simulink model "MCU_CmdTrans"  (R2022b)
settings: Solver=FixedStepDiscrete  StartTime=0.0  StopTime=10.0  FixedStep=0.001  RelTol=1e-3
undefined symbols (not defined in the file or in its folder): ANALOG, cAgeingMode, cCurrentLoopMode, cNoneMode, cParaRecogMode, cSingleBoardMode, cSpeedLoopMode, cTorqueLoopMode, cVvvfOpenMode, FAULT, ParamCfg_CommandSource_u16, ParamCfg_MaxSpeed_u16, ParamCfg_MaxTorque_u16, ParamCfg_Spdouttype_u16, ParamCfg_Vc1Enable_u16, POWER_ON, STANDBY, TESTBED, VEHICLE, WORKING
libraries: simulink x9
(part 2 of 2)

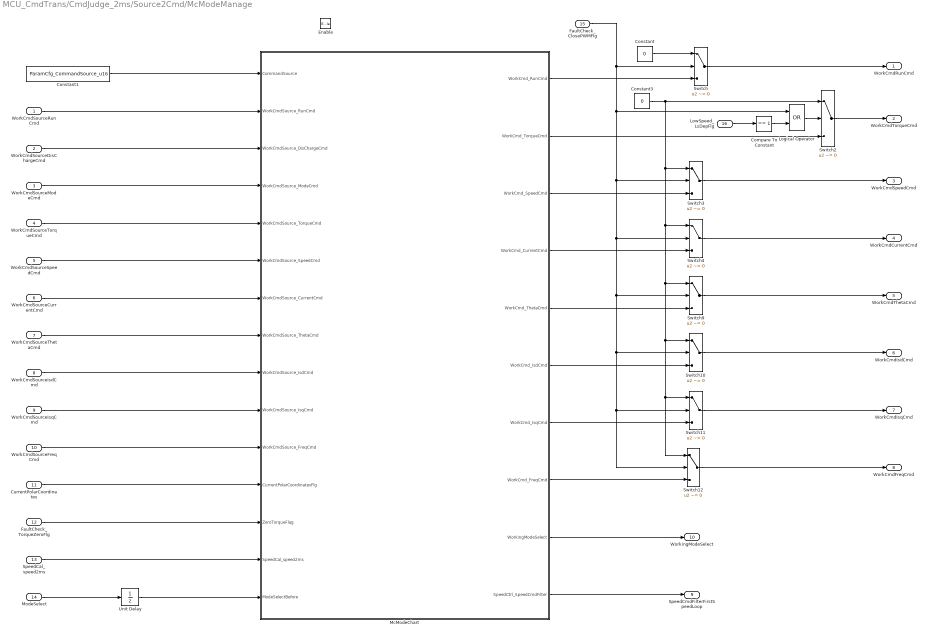
== system MCU_CmdTrans/CmdJudge_2ms/Source2Cmd/McModeManage ==
  WorkCmdSourceRunCmd : Inport
  WorkCmdSourceDisChargeCmd : Inport  Port=2
  WorkCmdSourceModeCmd : Inport  Port=3
  WorkCmdSourceTorqueCmd : Inport  Port=4
  WorkCmdSourceSpeedCmd : Inport  Port=5
  WorkCmdSourceCurrentCmd : Inport  Port=6
  WorkCmdSourceThetaCmd : Inport  Port=7
  WorkCmdSourceIsdCmd : Inport  Port=8
  WorkCmdSourceIsqCmd : Inport  Port=9
  WorkCmdSourceFreqCmd : Inport  Port=10
  CurrentPolarCoordinates : Inport  Port=11
  FaultCheck_TorqueZeroFlg : Inport  Port=12
  SpeedCal_speed2ms : Inport  Port=13
  ModeSelect : Inport  Port=14
  FaultCheck_ClosePWMFlg : Inport  Port=15
  LowSpeed_LsDepFlg : Inport  Port=16
  Enable : EnablePort
  Compare To Constant : simulink/Logic and Bit Operations/Compare To Constant  relop===  const=1  OutDataTypeStr=boolean
  Constant : Constant  Value=0  OutDataTypeStr=uint16
  Constant1 : Constant  Value=ParamCfg_CommandSource_u16
  Constant3 : Constant  Value=0  OutDataTypeStr=single
  Logical Operator : Logic  Operator=OR  AllPortsSameDT=off  OutDataTypeStr=boolean
  McModeChart : Stateflow chart  TreatAsAtomicUnit=on
      settings: FunctionInterfaceSpec=Allow arguments (Optimized)  PortSchema="{\"entries\":[{\"content\":{\"sides\":[{\"content\":{\"connectorIds\":[\"In2\",\"In5\",\"In3\",\"In4\",\"In6\",\"In11\",\"In7\",\"In1\",\"In9\",\"In10\",\"In8\",\"In12\",\"In13\",\"In14\",\"In15\"]},\"type\":\"ConnectorPlacement.EquallySpacedRectSide\",\"uuid\":\"2e7d3842-0a61-4590-9292-7a5bc1b6d63e\"},{\"content\":{\"connectorIds\":[\"Out2\",\"Out3\",\"Out4\",\"Out6\",\"Out5\",\"Out7\",\"Out8\",\"Out9\",\"Out1\",\"Out10\"],\"side\":\"RIGHT\"},\"type\":\"ConnectorPlacement.EquallySpacedRectSide\",\"uuid\":\"fb66f02a-321f-47a6-a489-4b94442e22c8\"},{\"content\":{\"connectorIds\":[],\"side\":\"TOP\"},\"type\":\"ConnectorPlacement.EquallySpacedRectSide\",\"uuid\":\"26cfdcf8-827e-48d9-aa42-40739db869be\"},{\"content\":{\"connectorIds\":[],\"side\":\"BOTTOM\"},\"type\":\"ConnectorPlacement.EquallySpacedRectSide\",\"uuid\":\"3bc2be8d-756f-48d1-976e-919451ea6fa2\"}]},\"type\":\"ConnectorPlacement.EquallySpacedConnector\",\"uuid\":\"eb156a25-beb1-4594-a414-e9203ec852c3\"}],\"packageUris\":[\"http://schema.mathworks.com/mf0/Connector/R2020b\"],\"version\":\"1.0\"}"
  Switch{,2..4,9..12} (8 alike) : Switch  Criteria=u2 ~= 0  SaturateOnIntegerOverflow=off  InputSameDT=off
  Unit Delay : UnitDelay  SampleTime=-1  HasFrameUpgradeWarning=on
  WorkCmdRunCmd : Outport
  WorkCmdTorqueCmd : Outport  Port=2
  WorkCmdSpeedCmd : Outport  Port=3
  WorkCmdCurrentCmd : Outport  Port=4
  WorkCmdThetaCmd : Outport  Port=5
  WorkCmdIsdCmd : Outport  Port=6
  WorkCmdIsqCmd : Outport  Port=7
  WorkCmdFreqCmd : Outport  Port=8
  SpeedCmdFilterFirstSpeedLoop : Outport  Port=9
  WorkingModeSelect : Outport  Port=10
  wires:
  Constant1/1 -> McModeChart/2(CommandSource)
  WorkCmdSourceRunCmd/1 -> McModeChart/5(WorkCmdSource_RunCmd)
  WorkCmdSourceModeCmd/1 -> McModeChart/4(WorkCmdSource_ModeCmd)
  WorkCmdSourceTorqueCmd/1 -> McModeChart/6(WorkCmdSource_TorqueCmd)
  WorkCmdSourceDisChargeCmd/1 -> McModeChart/3(WorkCmdSource_DisChargeCmd)
  WorkCmdSourceSpeedCmd/1 -> McModeChart/11(WorkCmdSource_SpeedCmd)
  WorkCmdSourceCurrentCmd/1 -> McModeChart/7(WorkCmdSource_CurrentCmd)
  WorkCmdSourceThetaCmd/1 -> McModeChart/1(WorkCmdSource_ThetaCmd)
  WorkCmdSourceIsdCmd/1 -> McModeChart/9(WorkCmdSource_IsdCmd)
  WorkCmdSourceIsqCmd/1 -> McModeChart/10(WorkCmdSource_IsqCmd)
  WorkCmdSourceFreqCmd/1 -> McModeChart/8(WorkCmdSource_FreqCmd)
  CurrentPolarCoordinates/1 -> McModeChart/12(CurrentPolarCoordinatesFlg)
  FaultCheck_TorqueZeroFlg/1 -> McModeChart/13(ZeroTorqueFlag)
  SpeedCal_speed2ms/1 -> McModeChart/14(SpeedCal_speed2ms)
  ModeSelect/1 -> Unit Delay/1
  Unit Delay/1 -> McModeChart/15(ModeSelectBefore)
  FaultCheck_ClosePWMFlg/1 -> Switch12/2, Switch11/2, Switch10/2, Switch9/2, Switch4/2, Switch3/2, Logical Operator/1, Switch/2
  McModeChart/2(WorkCmd_RunCmd) -> Switch/3
  Constant/1 -> Switch/1
  McModeChart/3(WorkCmd_TorqueCmd) -> Switch2/3
  Constant3/1 -> Switch12/1, Switch11/1, Switch10/1, Switch9/1, Switch4/1, Switch3/1, Switch2/1
  McModeChart/4(WorkCmd_SpeedCmd) -> Switch3/3
  McModeChart/6(WorkCmd_CurrentCmd) -> Switch4/3
  McModeChart/5(WorkCmd_ThetaCmd) -> Switch9/3
  McModeChart/7(WorkCmd_IsdCmd) -> Switch10/3
  McModeChart/8(WorkCmd_IsqCmd) -> Switch11/3
  McModeChart/9(WorkCmd_FreqCmd) -> Switch12/3
  McModeChart/10(SpeedCtrl_SpeedCmdFilter) -> SpeedCmdFilterFirstSpeedLoop/1
  Switch/1 -> WorkCmdRunCmd/1
  Switch2/1 -> WorkCmdTorqueCmd/1
  Switch3/1 -> WorkCmdSpeedCmd/1
  Switch4/1 -> WorkCmdCurrentCmd/1
  Switch9/1 -> WorkCmdThetaCmd/1
  Switch10/1 -> WorkCmdIsdCmd/1
  Switch11/1 -> WorkCmdIsqCmd/1
  Switch12/1 -> WorkCmdFreqCmd/1
  McModeChart/1(WorkingModeSelect) -> WorkingModeSelect/1
  LowSpeed_LsDepFlg/1 -> Compare To Constant/1
  Logical Operator/1 -> Switch2/2
  Compare To Constant/1 -> Logical Operator/2

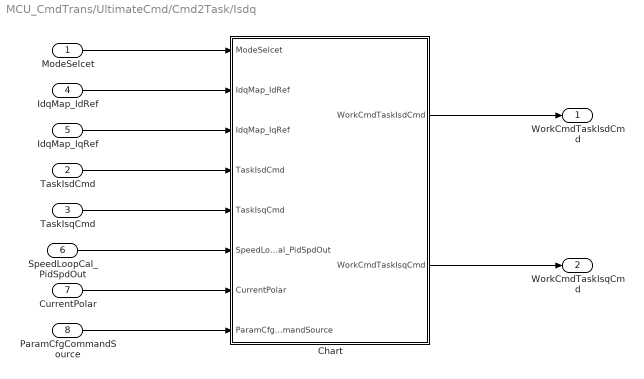
== system MCU_CmdTrans/UltimateCmd/Cmd2Task/Isdq ==
  ModeSelcet : Inport
  TaskIsdCmd : Inport  Port=2
  TaskIsqCmd : Inport  Port=3
  IdqMap_IdRef : Inport  Port=4
  IdqMap_IqRef : Inport  Port=5
  SpeedLoopCal_PidSpdOut : Inport  Port=6
  CurrentPolar : Inport  Port=7
  ParamCfgCommandSource : Inport  Port=8
  Chart : Stateflow chart  TreatAsAtomicUnit=on
  WorkCmdTaskIsdCmd : Outport
  WorkCmdTaskIsqCmd : Outport  Port=2
  wires:
  ModeSelcet/1 -> Chart/1(ModeSelcet)
  IdqMap_IdRef/1 -> Chart/2(IdqMap_IdRef)
  TaskIsdCmd/1 -> Chart/4(TaskIsdCmd)
  IdqMap_IqRef/1 -> Chart/3(IdqMap_IqRef)
  TaskIsqCmd/1 -> Chart/5(TaskIsqCmd)
  Chart/1(WorkCmdTaskIsdCmd) -> WorkCmdTaskIsdCmd/1
  Chart/2(WorkCmdTaskIsqCmd) -> WorkCmdTaskIsqCmd/1
  SpeedLoopCal_PidSpdOut/1 -> Chart/6(SpeedLoopCal_PidSpdOut)
  CurrentPolar/1 -> Chart/7(CurrentPolar)
  ParamCfgCommandSource/1 -> Chart/8(ParamCfgCommandSource)

== stateflow chart MCU_CmdTrans/UltimateCmd/Cmd2Task/Cmd2TaskChart ==
  (default) -> (junction 18)
  (junction 18) -> (junction 20) [order 1] : [WorkState_ModeSelect ==cTorqueLoopMode]
  (junction 18) -> (junction 50) [order 2]
  (junction 20) -> (junction 22) : {
      | WorkCmdTaskRunCmd = WorkCmdRunCmd;
      | WorkCmdTaskTorqueCmd = WorkCmdTorqueCmd;
      | }
  (junction 28) -> (junction 32) [order 1] : [(SpeedCal_HighSpdZeroTrqFlg == 0)&&(TorqeCtrl_TorqueCmdFilterAbs<0.001 && WorkCmdTaskTorqueCmd < 0.001)]{WorkCmdTaskRunCmd = STOP}
  (junction 22) -> (junction 25) [order 1] : [WorkCmdTaskTorqueCmd > 0]{SpeedCmdDir =1}
  (junction 22) -> (junction 25) [order 2] : {SpeedCmdDir = -1}
  (junction 25) -> (junction 28) : {WorkCmdTaskSpeedCmd = ParamCfg_MaxSpeed_u16 * SpeedCmdDir}
  (junction 28) -> (junction 32) [order 2]
  (junction 32) -> (junction 58)
  (junction 50) -> (junction 52) [order 1] : [WorkState_ModeSelect == cSpeedLoopMode]
  (junction 50) -> (junction 61) [order 2]
  (junction 52) -> (junction 54) : {WorkCmdTaskRunCmd = WorkCmdRunCmd;
      | WorkCmdTaskSpeedCmd = WorkCmdSpeedCmd;
      | WorkCmdTaskTorqueCmd = (ParamCfg_MaxTorque_u16 * 0.1)}
  (junction 54) -> (junction 58)
  (junction 58) -> (junction 67)
  (junction 61) -> (junction 63) [order 1] : [WorkState_ModeSelect == cCurrentLoopMode ]
  (junction 61) -> (junction 78) [order 2]
  (junction 63) -> (junction 65) : {WorkCmdTaskRunCmd = WorkCmdRunCmd}
  (junction 71) -> (junction 67) [order 1] : [(CurrentPolar == 1)&&ParamCfg_CommandSource_u16 == TESTBED]...
      | {WorkCmdTaskCurrentCmd = WorkCmdCurrentCmd;
      | WorkCmdTaskThetaCmd = WorkCmdThetaCmd;
      | WorkCmdTaskIsdCmd = WorkCmdTaskCurrentCmd * cos(WorkCmdTaskThetaCmd)*(-1)
      | WorkCmdTaskIsqCmd = WorkCmdTaskCurrentCmd * sin(WorkCmdTaskThetaCmd)
      | }
  (junction 71) -> (junction 67) [order 2] : {WorkCmdTaskIsdCmd = WorkCmdIsdCmd;
      | WorkCmdTaskIsqCmd = WorkCmdIsqCmd}
  (junction 65) -> (junction 71)
  (junction 67) -> (junction 85)
  (junction 78) -> (junction 80) [order 1] : [WorkState_ModeSelect == cVvvfOpenMode ]
  (junction 78) -> (junction 88) [order 2]
  (junction 80) -> (junction 83) : {WorkCmdTaskRunCmd = WorkCmdRunCmd;
      | WorkCmdTaskIsdCmd = WorkCmdIsdCmd;
      | WorkCmdTaskIsqCmd = WorkCmdIsqCmd;
      | WorkCmdTaskFreqCmd = WorkCmdFreqCmd;
      | }
  (junction 83) -> (junction 85)
  (junction 85) -> (junction 95)
  (junction 88) -> (junction 90) [order 1] : [WorkState_ModeSelect == cParaRecogMode ]
  (junction 88) -> (junction 98) [order 2]
  (junction 90) -> (junction 93) : {WorkCmdTaskRunCmd = WorkCmdRunCmd;
      | WorkCmdTaskRunCmd = WorkCmdRunCmd;
      | WorkCmdTaskIsdCmd = WorkCmdIsdCmd;
      | WorkCmdTaskIsqCmd = WorkCmdIsqCmd}
  (junction 93) -> (junction 95)
  (junction 95) -> (junction 105)
  (junction 98) -> (junction 100) [order 1] : [WorkState_ModeSelect == cSingleBoardMode ]
  (junction 98) -> (junction 108) [order 2]
  (junction 100) -> (junction 103) : {WorkCmdTaskRunCmd = WorkCmdRunCmd}
  (junction 103) -> (junction 105)
  (junction 105) -> (junction 125)
  (junction 108) -> (junction 110) [order 1] : [WorkState_ModeSelect == cAgeingMode ]
  (junction 108) -> (junction 112) [order 2]
  (junction 110) -> (junction 118) : {WorkCmdTaskRunCmd     = WorkCmdRunCmd;
      |  WorkCmdTaskCurrentCmd = (WorkCmdCurrentCmd);
      | WorkCmdTaskThetaCmd   = WorkCmdThetaCmd;
      |  WorkCmdTaskIsdCmd     = (WorkCmdTaskCurrentCmd * cos(WorkCmdTaskThetaCmd*2*PI));
      |  WorkCmdTaskIsqCmd     = (WorkCmdTaskCurrentCmd * sin(WorkCmdTaskThetaCmd*2*PI));
      |   WorkCmdTaskFreqCmd    = WorkCmdFreqCmd;}
  (junction 118) -> (junction 125)
  (junction 125) -> (junction 122)
  (junction 112) -> (junction 114) [order 1] : [WorkState_ModeSelect == cNoneMode ]
  (junction 112) -> (junction 129) [order 2]
  (junction 114) -> (junction 120) : {WorkCmdTaskRunCmd = STOP}
  (junction 120) -> (junction 122)
  (junction 122) -> (junction 131)
  (junction 131) -> (junction 129)
  (junction 129) -> (junction 134)
  data: WorkCmdIsdCmd input; WorkState_ModeSelect input; WorkCmdRunCmd input; WorkCmdTorqueCmd input; WorkCmdSpeedCmd input; WorkCmdCurrentCmd input; WorkCmdThetaCmd input; WorkCmdIsqCmd input; WorkCmdFreqCmd input; WorkCmdTaskRunCmd output uint16 =0; WorkCmdTaskTorqueCmd output single =0; WorkCmdTaskSpeedCmd output single =0; WorkCmdTaskCurrentCmd output single =0; WorkCmdTaskThetaCmd output single =0; WorkCmdTaskIsdCmd output single =0; WorkCmdTaskIsqCmd output single =0; WorkCmdTaskFreqCmd output single =0; cTorqueLoopMode parameter; SpeedCmdDir output double; SpeedCal_HighSpdZeroTrqFlg input; TorqeCtrl_TorqueCmdFilterAbs input; ParamCfg_MaxSpeed_u16 parameter; STOP constant uint16 =0; cSpeedLoopMode parameter; cCurrentLoopMode parameter; ParamCfg_MaxTorque_u16 parameter; CurrentPolar input; ParamCfg_CommandSource_u16 parameter; TESTBED parameter; cVvvfOpenMode parameter; cParaRecogMode parameter; cSingleBoardMode parameter; cAgeingMode parameter; cNoneMode parameter; PI constant single =3.141592

== stateflow chart MCU_CmdTrans/UltimateCmd/Cmd2Task/Isdq/Chart ==
  (default) -> (junction 8) : {
      | WorkCmdTaskIsdCmd = TaskIsdCmd;
      | WorkCmdTaskIsqCmd = TaskIsqCmd;
      | }
  (junction 8) -> (junction 10) [order 1] : [(ModeSelcet == cTorqueLoopMode) || (ModeSelcet==cSpeedLoopMode && ParamCfg_Spdouttype_u16 == 0)]
      | {WorkCmdTaskIsdCmd = IdqMap_IdRef;
      | WorkCmdTaskIsqCmd  = IdqMap_IqRef}
  (junction 8) -> (junction 10) [order 2]
  (junction 10) -> (junction 18) [order 1] : [ModeSelcet == cSpeedLoopMode &&ParamCfg_Spdouttype_u16 ==1 ]
      | {
      | WorkCmdTaskIsdCmd = 0;
      | WorkCmdTaskIsqCmd = SpeedLoopCal_PidSpdOut;
      | }
  (junction 10) -> (junction 18) [order 2]
  (junction 18) -> (junction 22) [order 1] : [ModeSelcet == cCurrentLoopMode && CurrentPolar == 1 && ParamCfgCommandSource == TESTBED]
      | {
      | WorkCmdTaskIsdCmd = 0;
      | WorkCmdTaskIsqCmd = SpeedLoopCal_PidSpdOut;
      | }
  (junction 18) -> (junction 22) [order 2]
  (junction 22) -> (junction 29)
  data: ModeSelcet input; IdqMap_IdRef input single; IdqMap_IqRef input single; TaskIsdCmd input; TaskIsqCmd input; WorkCmdTaskIsdCmd output; WorkCmdTaskIsqCmd output; cSpeedLoopMode parameter; cTorqueLoopMode parameter; ParamCfg_Spdouttype_u16 parameter; SpeedLoopCal_PidSpdOut input single; cCurrentLoopMode parameter; CurrentPolar input; ParamCfgCommandSource input; TESTBED parameter

== stateflow chart MCU_CmdTrans/CmdJudge_2ms/CAN2Source/Chart ==
  (default) -> (junction 26) : {
      | WorkCmdSourceRunCmd = RunCmd;
      | WorkCmdSourceDisChargeCmd = DisChargeCmd;
      | WorkCmdSourceModeCmd = ModeCmd;
      | WorkCmdSourceTorqueCmd = TorqueCmd;
      | WorkCmdSourceSpeedCmd = SpeedCmd;
      | WorkCmdSourceCurrentCmd = CurrentCmd;
      | WorkCmdSourceThetaCmd = ThetaCmd;
      | WorkCmdSourceIsdCmd = IsdCmd;
      | WorkCmdSourceIsqCmd = IsqCmd;
      | WorkCmdSourceFreqCmd = FreqCmd;
      | }
  (junction 26) -> (junction 28) [order 1] : [LsDepFlg == 1]{WorkCmdSourceTorqueCmd=0}
  (junction 26) -> (junction 28) [order 2]
  (junction 28) -> (junction 31) [order 1] : [FaultCheck_LostPhaseFaultFlg == 1]...
      | {WorkCmdSourceRunCmd = 1;
      | WorkCmdSourceModeCmd = cTorqueLoopMode}
  (junction 28) -> (junction 31) [order 2]
  (junction 31) -> (junction 35) [order 2] : [ActDisChargeStd == 1]...
      | {WorkCmdSourceRunCmd = 1;
      | WorkCmdSourceModeCmd = cCurrentLoopMode;
      | WorkCmdSourceIsdCmd = ActDisChargeCurr;
      | WorkCmdSourceIsqCmd = 0;
      | CurrentPolarCoordinates =0;}
  (junction 31) -> (junction 35) [order 1]
  (junction 35) -> (junction 40)
  data: RunCmd input; WorkCmdSourceRunCmd output uint16 =0; WorkCmdSourceDisChargeCmd output uint16 =0; WorkCmdSourceModeCmd output uint16 =0; WorkCmdSourceTorqueCmd output single =0; WorkCmdSourceSpeedCmd output single =0; WorkCmdSourceCurrentCmd output single =0; WorkCmdSourceThetaCmd output single =0; WorkCmdSourceIsdCmd output single =0; WorkCmdSourceIsqCmd output single =0; WorkCmdSourceFreqCmd output single =0; DisChargeCmd input; ModeCmd input; TorqueCmd input; SpeedCmd input; CurrentCmd input; ThetaCmd input; IsdCmd input; IsqCmd input; FreqCmd input; ActDisChargeStd input; ActDisChargeCurr input; FaultCheck_LostPhaseFaultFlg input; LsDepFlg input; cTorqueLoopMode parameter; cCurrentLoopMode parameter; CurrentPolarCoordinates output uint16 =0

== stateflow chart MCU_CmdTrans/CmdJudge_2ms/Source2Cmd/McModeManage/McModeChart ==
  (default) -> (junction 10)
  (junction 267) -> (junction 270) [order 1] : [WorkCmdSource_ModeCmd==cTorqueLoopMode]
  (junction 265) -> (junction 267) : [CommandSource == VEHICLE]
  (junction 10) -> (junction 265) [order 2]
  (junction 10) -> (junction 12) [order 1] : [CommandSource == TESTBED]
  (junction 12) -> (junction 40) [order 1] : [WorkCmdSource_ModeCmd==cTorqueLoopMode]
  (junction 270) -> (junction 344) : {WorkingModeSelect = cTorqueLoopMode;
      | WorkCmd_RunCmd = WorkCmdSource_RunCmd;
      | WorkCmd_TorqueCmd = WorkCmdSource_TorqueCmd;}
  (junction 267) -> (junction 274) [order 2]
  (junction 10) -> (junction 289) [order 3] : [CommandSource == ANALOG]
  (junction 12) -> (junction 47) [order 2]
  (junction 40) -> (junction 43) : {WorkingModeSelect = cTorqueLoopMode;
      | WorkCmd_RunCmd = WorkCmdSource_RunCmd;
      | WorkCmd_TorqueCmd = WorkCmdSource_TorqueCmd;}
  (junction 43) -> (junction 243)
  (junction 243) -> (junction 238)
  (junction 47) -> (junction 49) [order 1] : [WorkCmdSource_ModeCmd ==cSpeedLoopMode ]
  (junction 47) -> (junction 57) [order 2]
  (junction 49) -> (junction 54) : {WorkingModeSelect = cSpeedLoopMode;
      | WorkCmd_RunCmd = WorkCmdSource_RunCmd;
      | WorkCmd_SpeedCmd = WorkCmdSource_SpeedCmd;}
  (junction 274) -> (junction 337) [order 1] : [WorkCmdSource_ModeCmd ==cSpeedLoopMode]
  (junction 337) -> (junction 342) : {WorkingModeSelect = cSpeedLoopMode;
      | WorkCmd_RunCmd = WorkCmdSource_RunCmd;
      | }
  (junction 274) -> (junction 347) [order 2]
  (junction 328) -> (junction 238) [order 1] : [ModeSelectBefore ~= cSpeedLoopMode]{SpeedCtrl_SpeedCmdFilter = SpeedCal_speed2ms}
  (junction 289) -> (junction 292)
  (junction 342) -> (junction 344) [order 1] : [ModeSelectBefore ~= cSpeedLoopMode]{SpeedCtrl_SpeedCmdFilter = SpeedCal_speed2ms}
  (junction 54) -> (junction 328)
  (junction 328) -> (junction 238) [order 2]
  (junction 238) -> (junction 233)
  (junction 342) -> (junction 344) [order 2]
  (junction 292) -> (junction 296) [order 1] : [WorkCmdSource_ModeCmd == cTorqueLoopMode]
  (junction 344) -> (junction 353)
  (junction 292) -> (junction 302) [order 2]
  (junction 296) -> (junction 298) : {WorkingModeSelect = cTorqueLoopMode;
      | WorkCmd_RunCmd = WorkCmdSource_RunCmd;
      | WorkCmd_TorqueCmd = WorkCmdSource_TorqueCmd;}
  (junction 57) -> (junction 59) [order 1] : [WorkCmdSource_ModeCmd ==cCurrentLoopMode ]
  (junction 57) -> (junction 78) [order 2]
  (junction 59) -> (junction 61) : {WorkingModeSelect = cCurrentLoopMode;
      | WorkCmd_RunCmd = WorkCmdSource_RunCmd;}
  (junction 347) -> (junction 349) [order 1] : [WorkCmdSource_ModeCmd ==cCurrentLoopMode]
  (junction 349) -> (junction 351) : {WorkingModeSelect = cCurrentLoopMode;
      | WorkCmd_IsdCmd = WorkCmdSource_IsdCmd;
      | WorkCmd_IsqCmd = WorkCmdSource_IsqCmd}
  (junction 347) -> (junction 356) [order 2]
  (junction 61) -> (junction 64) [order 1] : [CurrentPolarCoordinatesFlg ==1]
  (junction 298) -> (junction 300)
  (junction 61) -> (junction 71) [order 2] : {WorkCmd_IsdCmd = WorkCmdSource_IsdCmd;
      | WorkCmd_IsqCmd = WorkCmdSource_IsqCmd}
  (junction 64) -> (junction 66) : {WorkCmd_CurrentCmd = WorkCmdSource_CurrentCmd;
      | WorkCmd_ThetaCmd = WorkCmdSource_ThetaCmd;}
  (junction 300) -> (junction 308)
  (junction 302) -> (junction 304) [order 1] : [WorkCmdSource_ModeCmd == cSpeedLoopMode]
  (junction 66) -> (junction 71)
  (junction 302) -> (junction 311) [order 2]
  (junction 304) -> (junction 306)
  (junction 71) -> (junction 74)
  (junction 351) -> (junction 353)
  (junction 332) -> (junction 308) [order 1] : [ModeSelectBefore ~= cSpeedLoopMode]{SpeedCtrl_SpeedCmdFilter = SpeedCal_speed2ms}
  (junction 353) -> (junction 364)
  (junction 74) -> (junction 233)
  (junction 233) -> (junction 228)
  (junction 306) -> (junction 332) : {WorkingModeSelect = cSpeedLoopMode;
      | WorkCmd_RunCmd = WorkCmdSource_RunCmd;
      | WorkCmd_TorqueCmd = WorkCmdSource_SpeedCmd;}
  (junction 332) -> (junction 308) [order 2]
  (junction 308) -> (junction 313)
  (junction 78) -> (junction 81) [order 1] : [WorkCmdSource_ModeCmd ==cVvvfOpenMode ]
  (junction 78) -> (junction 87) [order 2]
  (junction 81) -> (junction 83) : {WorkingModeSelect = cVvvfOpenMode;
      | WorkCmd_RunCmd = WorkCmdSource_RunCmd;
      | WorkCmd_FreqCmd = WorkCmdSource_FreqCmd;}
  (junction 356) -> (junction 360) [order 1] : [WorkCmdSource_ModeCmd ==cNoneMode]
  (junction 360) -> (junction 362) : {WorkingModeSelect = cNoneMode;
      | WorkCmd_RunCmd = WorkCmdSource_RunCmd;}
  (junction 356) -> (junction 367) [order 2] : {WorkingModeSelect = cNoneMode;}
  (junction 83) -> (junction 228)
  (junction 228) -> (junction 223)
  (junction 313) -> (junction 311)
  (junction 311) -> (junction 317) [order 2]
  (junction 311) -> (junction 317) [order 1] : [ZeroTorqueFlag == 1]
      | {WorkingModeSelect = cTorqueLoopMode;
      | WorkCmd_RunCmd = WorkCmdSource_RunCmd;
      | WorkCmd_TorqueCmd = 0;}
  (junction 87) -> (junction 89) [order 1] : [WorkCmdSource_ModeCmd ==cParaRecogMode ]
  (junction 87) -> (junction 94) [order 2]
  (junction 89) -> (junction 91) : {WorkingModeSelect = cParaRecogMode;
      | WorkCmd_RunCmd = WorkCmdSource_RunCmd;}
  (junction 362) -> (junction 364)
  (junction 364) -> (junction 369)
  (junction 367) -> (junction 371)
  (junction 317) -> (junction 319)
  (junction 91) -> (junction 223)
  (junction 223) -> (junction 252)
  (junction 94) -> (junction 96) [order 1] : [WorkCmdSource_ModeCmd ==cSingleBoardMode ]
  (junction 94) -> (junction 100) [order 2]
  (junction 96) -> (junction 98) : {WorkingModeSelect = cSingleBoardMode;
      | WorkCmd_RunCmd = WorkCmdSource_RunCmd;}
  (junction 369) -> (junction 371)
  (junction 371) -> (junction 374) [order 2]
  (junction 371) -> (junction 374) [order 1] : [ZeroTorqueFlag == 1]
      | {WorkingModeSelect = cTorqueLoopMode;
      | WorkCmd_RunCmd = WorkCmdSource_RunCmd;
      | WorkCmd_TorqueCmd = 0;}
  (junction 98) -> (junction 252)
  (junction 252) -> (junction 254)
  (junction 100) -> (junction 102) [order 1] : [WorkCmdSource_ModeCmd ==cAgeingMode ]
  (junction 100) -> (junction 108) [order 2]
  (junction 102) -> (junction 104) : {WorkingModeSelect = cAgeingMode;
      | WorkCmd_RunCmd = WorkCmdSource_RunCmd;
      | WorkCmd_CurrentCmd = WorkCmdSource_CurrentCmd;
      | WorkCmd_ThetaCmd = WorkCmdSource_ThetaCmd;
      | WorkCmd_FreqCmd = WorkCmdSource_FreqCmd;}
  (junction 104) -> (junction 254)
  (junction 374) -> (junction 375)
  (junction 254) -> (junction 256)
  (junction 108) -> (junction 110) [order 1] : [WorkCmdSource_ModeCmd ==cNoneMode ]
  (junction 108) -> (junction 262) [order 2] : {WorkingModeSelect = cNoneMode;}
  (junction 110) -> (junction 112) : {WorkingModeSelect = cNoneMode;
      | WorkCmd_RunCmd = WorkCmdSource_RunCmd;}
  (junction 112) -> (junction 256)
  (junction 256) -> (junction 260)
  (junction 260) -> (junction 262)
  (junction 262) -> (junction 259)
  (junction 259) -> (junction 280) [order 2]
  (junction 259) -> (junction 280) [order 1] : [ZeroTorqueFlag == 1]
      | {WorkingModeSelect = cTorqueLoopMode;
      | WorkCmd_RunCmd = WorkCmdSource_RunCmd;
      | WorkCmd_TorqueCmd = 0;}
  (junction 280) -> (junction 324)
  data: WorkCmdSource_ThetaCmd input; CommandSource input; WorkCmdSource_DisChargeCmd input; WorkCmdSource_ModeCmd input; WorkCmdSource_RunCmd input; WorkCmdSource_TorqueCmd input; WorkCmdSource_CurrentCmd input; WorkCmdSource_FreqCmd input; WorkCmdSource_IsdCmd input; WorkCmdSource_IsqCmd input; WorkCmdSource_SpeedCmd input; TESTBED parameter; cTorqueLoopMode parameter; WorkingModeSelect output uint16 =cNoneMode; cSpeedLoopMode parameter; WorkCmd_RunCmd output uint16 =0; WorkCmd_TorqueCmd output single =0; WorkCmd_SpeedCmd output single =0; cCurrentLoopMode parameter; WorkCmd_ThetaCmd output single =0; WorkCmd_CurrentCmd output single =0; CurrentPolarCoordinatesFlg input; WorkCmd_IsdCmd output single =0; WorkCmd_IsqCmd output single =0; cVvvfOpenMode parameter; WorkCmd_FreqCmd output single =0; cParaRecogMode parameter; cAgeingMode parameter; cSingleBoardMode parameter; cNoneMode parameter; VEHICLE parameter; ZeroTorqueFlag input; SpeedCal_speed2ms input; ANALOG parameter; ModeSelectBefore input; SpeedCtrl_SpeedCmdFilter output single =0

== stateflow chart MCU_CmdTrans/UltimateCmd/Task2Core/Chart ==
  (default) -> (junction 7) : {WorkCmdCoreRunCmd = WorkCmdTaskCmdRunCmd;
      | WorkCmdCoreModeCmd = ModeSelcet}
  (junction 7) -> (junction 11) [order 1] : [ParamCfg_Vc1Enable_u16 == 1 && ModeSelcet ==cTorqueLoopMode || (ModeSelcet ==cCurrentLoopMode && ParamCfg_CommandSource_u16 == TESTBED)]
  (junction 7) -> (junction 20) [order 2] : {WorkCmdCoreIsdCmd = WorkCmdTaskIsdCmd;
      | WorkCmdCoreIsqCmd = WorkCmdTaskIsqCmd;}
  (junction 11) -> (junction 18) : {WorkCmdCoreIsdCmd=VoltLoop_IdOut
      | WorkCmdCoreIsqCmd = VoltLoop_IqOut}
  (junction 18) -> (junction 20)
  (junction 20) -> (junction 26) : {WorkCmdCoreCurrentCmd = sqrt(WorkCmdCoreIsdCmd * WorkCmdCoreIsdCmd + WorkCmdCoreIsqCmd * WorkCmdCoreIsqCmd)}
  data: ModeSelcet input; WorkCmdTaskIsdCmd input; WorkCmdTaskIsqCmd input; VoltLoop_IdOut input single; VoltLoop_IqOut input single; ParamCfg_Vc1Enable_u16 parameter; WorkCmdTaskCmdRunCmd input; WorkCmdCoreRunCmd output; cTorqueLoopMode parameter; WorkCmdCoreModeCmd output; cCurrentLoopMode parameter; TESTBED parameter; ParamCfg_CommandSource_u16 parameter; WorkCmdCoreIsdCmd output single; WorkCmdCoreIsqCmd output single; WorkCmdCoreCurrentCmd output
